simulink model "sf_semantics_hotel_checkin"  (R2017b)
settings: Solver=FixedStepDiscrete  StartTime=0.0  StopTime=Inf  FixedStep=0.2  RelTol=1e-3  EnableMultiTasking=on
settings Model: Creator=The MathWorks, Inc.  LastModifiedBy=The MathWorks, Inc.
settings DataIOCC: LimitDataPoints=on  SaveCompleteFinalSimState=on  SaveFormat=Array
settings OptimizationCC: ExpressionDepthLimit=2147483647  InitFltsAndDblsToZero=on  LifeSpan=inf
settings DebuggingCC: UnderspecifiedInitializationDetection=Classic  MergeDetectMultiDrivingBlocksExec=none  SolverPrmCheckMsg=warning  FcnCallInpInsideContextMsg=warning  StateNameClashWarn=warning  SFUnexpectedBacktrackingDiag=warning  SFNoUnconditionalDefaultTransitionDiag=warning  SFExecutionAtInitializationDiag=none
settings HardwareCC: ProdBitPerPointer=32  ProdBitPerSizeT=32  ProdBitPerPtrDiffT=32  ProdLargestAtomicFloat=None  ProdIntDivRoundTo=Undefined  ProdEndianess=Unspecified  ProdWordSize=32  ProdHWDeviceType=32-bit Generic
settings ModelReferenceCC: PropagateSignalLabelsOutOfModel=off
settings SFSimCC: SimParseCustomCode=off
settings RTWCC: GenerateReport=on  LaunchReport=on
settings CodeAppCC: StateflowObjectComments=on
settings GRTTargetCC: TargetLangStandard=C89/C90 (ANSI)  GeneratePreprocessorConditionals=Disable all  CombineOutputUpdateFcns=off  GRTInterface=on
settings ConfigComp: CovMetricSettings=dw  CovHtmlReporting=on  CovSaveCumulativeToWorkspaceVar=on  CovSaveSingleToWorkspaceVar=on  CovExternalEMLEnable=off  CovSFcnEnable=off

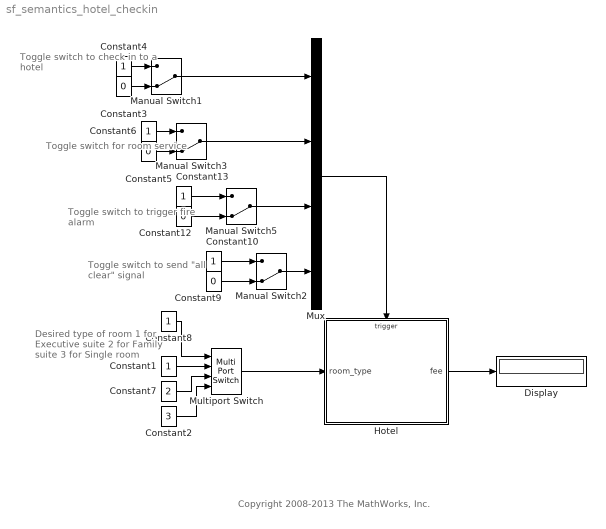
== system sf_semantics_hotel_checkin ==
  note: Desired type of room
      | 1 for Executive suite
      | 2 for Family suite
      | 3 for Single room
  note: Toggle switch to
      | check in to a hotel
  note: Toggle switch
      | for room service
  note: Toggle switch
      | to trigger fire alarm
  note: Toggle switch to
      | send "all clear" signal
  note: Copyright 2008-2013 The MathWorks, Inc.
  Constant{1,4,6,8,10,13} (6 alike) : Constant
  Constant{3,5,9,12} (4 alike) : Constant  Value=0
  Constant2 : Constant  Value=3
  Constant7 : Constant  Value=2
  Display : Display
  Hotel : Stateflow chart  TreatAsAtomicUnit=on
  Manual Switch{1..3,5} (4 alike) : ManualSwitch  CurrentSetting=0
  Multiport Switch : MultiPortSwitch
  Mux : Mux
  wires:
  Constant4/1 -> Manual Switch1/1
  Constant3/1 -> Manual Switch1/2
  Hotel/1(fee) -> Display/1
  Manual Switch1/1 -> Mux/1
  Manual Switch3/1 -> Mux/2
  Mux/1 -> Hotel/Trigger
  Multiport Switch/1 -> Hotel/1(room_type)
  Constant1/1 -> Multiport Switch/2
  Constant2/1 -> Multiport Switch/4
  Constant7/1 -> Multiport Switch/3
  Constant8/1 -> Multiport Switch/1
  Constant6/1 -> Manual Switch3/1
  Constant5/1 -> Manual Switch3/2
  Constant13/1 -> Manual Switch5/1
  Constant12/1 -> Manual Switch5/2
  Manual Switch5/1 -> Mux/3
  Constant10/1 -> Manual Switch2/1
  Constant9/1 -> Manual Switch2/2
  Manual Switch2/1 -> Mux/4

== stateflow chart sf_semantics_hotel_checkin/Hotel ==
  state Check_in
    (history)
    state Checked_in
      on room_service:
      service = service + 1;
      fee = expenses(service);
      (history)
      state Executive_suite
        (history)
        state Dining_area
        state Bedroom
        Bedroom -> Dining_area : room_service
        (default) -> Bedroom
        Dining_area -> Bedroom : room_service
      state Family_suite
        state Master_bedroom [parallel]
          settings: executionOrder=1
        state Second_bedroom [parallel]
          settings: executionOrder=2
      state Single_room
      (default) -> (junction 14) : {service=0;}
      (junction 14) -> Executive_suite [order 1] : [room_type == 1]  {fee = 1500;}
      (junction 14) -> (junction 26) [order 2]
      (junction 26) -> Family_suite [order 1] : [room_type == 2]  {fee = 1000;}
      (junction 26) -> (junction 129) [order 2]
      (junction 129) -> Single_room : [room_type == 3]  {fee = 500;}
    state Front_desk
    (default) -> Front_desk
    Front_desk -> Checked_in : check_in
  state Waiting_area
  (default) -> Check_in
  Check_in -> Waiting_area : fire_alarm
  Waiting_area -> Check_in : all_clear
  data: y function_output double; x function_input double; room_type input; fee output double; service local double
  events: check_in input EITHER_EDGE_EVENT; room_service input EITHER_EDGE_EVENT; fire_alarm input EITHER_EDGE_EVENT; all_clear input EITHER_EDGE_EVENT
  function y = expenses(x):
    | function y = expenses(x)
    | 
    | if (room_type == 1)
    |    y = 1500 + (x*50);    
    | else
    |    if (room_type == 2)
    |       y = 1000 + (x*25);
    |    else 
    |       y = 500 + (x*5);
    |    end
    | end
